simulink model "Clock"  (R2023a)
settings: Solver=VariableStepAuto  StartTime=0.0  StopTime=inf  MaxStep=1  MinStep=1  RelTol=1e-3  EnableMultiTasking=on
libraries: Counters_Lib x14, Nibble_Multiplexers_Lib x9, Bit_Multiplexers_Lib x9, simulink x6, simulink_extras x2, Decoders_Lib x1
settings Model: SimulationMode=accelerator  PauseTimes=0  NumberOfSteps=2  Creator=Jozko Mrkvicka  LastModifiedBy=Jozko Mrkvicka
settings SolverCC: InitialStep=1  AlgebraicLoopSolver=TrustRegion
settings DataIOCC: ReturnWorkspaceOutputs=off
settings OptimizationCC: LifeSpan=inf
settings DebuggingCC: UnconnectedInputMsg=warning  UnconnectedOutputMsg=warning  UnconnectedLineMsg=warning  SFUnexpectedBacktrackingDiag=warning  SFNoUnconditionalDefaultTransitionDiag=warning  ArithmeticOperatorsInVariantConditions=warning
settings ModelReferenceCC: EnableRefExpFcnMdlSchedulingChecks=on
settings SFSimCC: SimUseLocalCustomCode=off  CustomCodeUndefinedFunction=UseInterfaceOnly
settings RTWCC: RTWUseLocalCustomCode=off
settings CodeAppCC: StateflowObjectComments=on
settings GRTTargetCC: TargetLangStandard=C89/C90 (ANSI)
settings ConfigComp: CovMetricSettings=dw  CovSaveCumulativeToWorkspaceVar=on  CovSaveSingleToWorkspaceVar=on  CovExternalEMLEnable=off

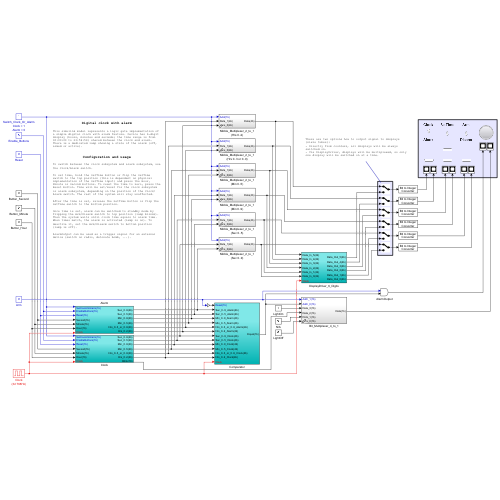
[thumbnail: Simulink's stored preview of the top-level diagram]
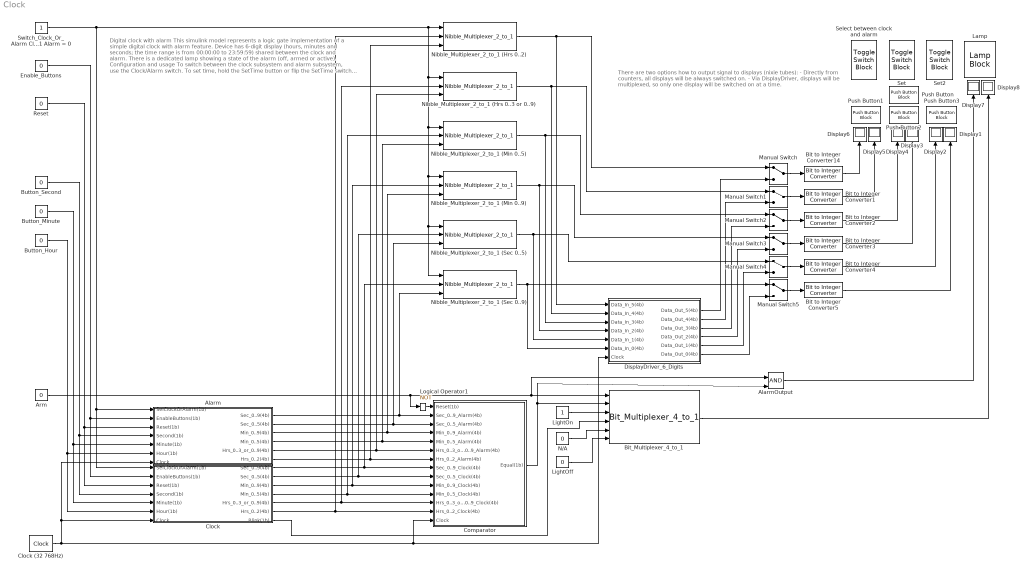
== system Clock ==
  note: There are two options how to output signal to displays (nixie tubes):
      | - Directly from counters, all displays will be always switched on.
      | - Via DisplayDriver, displays will be multiplexed, so only one display will be switched on at a time.
  note: Digital clock with alarm
      |
      | This simulink model represents a logic gate implementation of a simple digital clock with alarm feature. Device has 6-digit display (hours, minutes and seconds; the time range is from 00:00:00 to 23:59:59) shared between the clock and alarm. There is a dedicated lamp showing a state of the alarm (off, armed or active).
      |
      | Configuration and usage
      |
      | To switch between the clock subsystem and alarm subsystem, use the Clock/Alarm switch.
      |
      | To set time, hold the SetTime button or flip the SetTime switch to the top position (this is dependent on physical implementation of the SetTime input) and press the Hour, Minute or Second buttons. To reset the time to zero, press the Reset button. Time will be set/reset for the clock subsystem or alarm subsystem, depending on the position of the Clock/Alarm switch. The rest of the system will stay unaffected.
      |
      | After the time is set, release the SetTime button or flip the SetTime switch to the bottom position.
      |
      | Once time is set, alarm can be switched to standby mode by flipping the Arm/Disarm switch to top position (lamp blinks). Then the system waits until clock time equals to alarm time. When times match, the alarm is activated (lamp is on). To deactive it, set the Arm/Disarm switch to bottom position (lamp is off).
      |
      | AlarmOutput can be used as a trigger signal for an external device (switch on radio, detonate bomb, ...).
  Alarm : Subsystem
  AlarmOutput : Logic  IconShape=distinctive  AllPortsSameDT=off  OutDataTypeStr=boolean
  Arm : Constant  Value=0
  Bit to Integer Converter{1..5,14} (6 alike) : simulink/Logic and Bit Operations/Bit to Integer Converter  nbits=4  bitOrder=MSB first  signedOutputValues=Unsigned  outDtype=uint8  outDtypeSigned=Inherit via internal rule
      settings: LibrarySourceBlock=|
      | commutil2/Bit to Integer
      | Converter
  Bit_Multiplexer_4_to_1 : Bit_Multiplexers_Lib/Bit_Multiplexers_Lib/Bit_Multiplexer_4_to_1  SystemSampleTime=-1  VariantActivationTime=update diagram  Latency=0  AutoFrameSizeCalculation=off
  Button_Hour : Constant  Value=0
  Button_Minute : Constant  Value=0
  Button_Second : Constant  Value=0
  Clock : Subsystem
  Clock (32 768Hz) : simulink_extras/Flip Flops/Clock  period=1
  Comparator : Subsystem
  Display{1..8} (8 alike) : Display
  DisplayDriver_6_Digits : Subsystem
  Enable_Buttons : Constant  Value=0
  Lamp : LampBlock  LabelPosition=Hide
  LightOff : Constant  Value=0
  LightOn : Constant
  Logical Operator1 : Logic  Operator=NOT  Inputs=4  IconShape=distinctive  AllPortsSameDT=off  OutDataTypeStr=boolean
  Manual Switch{,1..5} (6 alike) : ManualSwitch
  N/A : Constant  Value=0
  Nibble_Multiplexer_2_to_1 (Hrs 0..2) : Nibble_Multiplexers_Lib/Nibble_Multiplexers_Lib/Nibble_Multiplexer_2_to_1  SystemSampleTime=-1  VariantActivationTime=update diagram  Latency=0  AutoFrameSizeCalculation=off
  Nibble_Multiplexer_2_to_1 (Hrs 0..3 or 0..9) : Nibble_Multiplexers_Lib/Nibble_Multiplexers_Lib/Nibble_Multiplexer_2_to_1  SystemSampleTime=-1  VariantActivationTime=update diagram  Latency=0  AutoFrameSizeCalculation=off
  Nibble_Multiplexer_2_to_1 (Min 0..5) : Nibble_Multiplexers_Lib/Nibble_Multiplexers_Lib/Nibble_Multiplexer_2_to_1  SystemSampleTime=-1  VariantActivationTime=update diagram  Latency=0  AutoFrameSizeCalculation=off
  Nibble_Multiplexer_2_to_1 (Min 0..9) : Nibble_Multiplexers_Lib/Nibble_Multiplexers_Lib/Nibble_Multiplexer_2_to_1  SystemSampleTime=-1  VariantActivationTime=update diagram  Latency=0  AutoFrameSizeCalculation=off
  Nibble_Multiplexer_2_to_1 (Sec 0..5) : Nibble_Multiplexers_Lib/Nibble_Multiplexers_Lib/Nibble_Multiplexer_2_to_1  SystemSampleTime=-1  VariantActivationTime=update diagram  Latency=0  AutoFrameSizeCalculation=off
  Nibble_Multiplexer_2_to_1 (Sec 0..9) : Nibble_Multiplexers_Lib/Nibble_Multiplexers_Lib/Nibble_Multiplexer_2_to_1  SystemSampleTime=-1  VariantActivationTime=update diagram  Latency=0  AutoFrameSizeCalculation=off
  Push Button : PushButtonBlock  ButtonText=Reset
  Push Button1 : PushButtonBlock  ButtonText=Hour  OffValue=0.000000
  Push Button2 : PushButtonBlock  ButtonText=Minute  OffValue=0.000000
  Push Button3 : PushButtonBlock  ButtonText=Second
  Reset : Constant  Value=0
  Select between clock and alarm : ToggleSwitchBlock  LabelPosition=Hide
      settings: Values={{'Alarm', 'Clock'}, [0 1]}
  Set : ToggleSwitchBlock  LabelPosition=Hide
      settings: Values={{' ', 'SetTime'}, [0 1]}
  Set2 : ToggleSwitchBlock  LabelPosition=Hide
      settings: Values={{'Disarm', 'Arm'}, [0 1]}
  Switch_Clock_Or_Alarm Clock = 1 Alarm = 0 : Constant
  wires:
  Clock (32 768Hz)/1 -> DisplayDriver_6_Digits/7(Clock), Comparator/14(Clock), Clock/7(Clock), Alarm/7(Clock)
  Enable_Buttons/1 -> Clock/2(EnableButtons(1b)), Alarm/2(EnableButtons(1b))
  Reset/1 -> Clock/3(Reset(1b)), Alarm/3(Reset(1b))
  Switch_Clock_Or_Alarm Clock = 1 Alarm = 0/1 -> Nibble_Multiplexer_2_to_1 (Sec 0..9)/1, Nibble_Multiplexer_2_to_1 (Sec 0..5)/1, Nibble_Multiplexer_2_to_1 (Min 0..9)/1, Nibble_Multiplexer_2_to_1 (Min 0..5)/1, Nibble_Multiplexer_2_to_1 (Hrs 0..3 or 0..9)/1, Nibble_Multiplexer_2_to_1 (Hrs 0..2)/1, Clock/1(SelClockOrAlarm(1b)), Alarm/1(SelClockOrAlarm(1b))
  Button_Hour/1 -> Clock/6(Hour(1b)), Alarm/6(Hour(1b))
  Button_Minute/1 -> Clock/5(Minute(1b)), Alarm/5(Minute(1b))
  Button_Second/1 -> Clock/4(Second(1b)), Alarm/4(Second(1b))
  Alarm/6(Hrs_0..2(4b)) -> Nibble_Multiplexer_2_to_1 (Hrs 0..2)/3, Comparator/7(Hrs_0..2_Alarm(4b))
  Alarm/5(Hrs_0..3_or_0..9(4b)) -> Nibble_Multiplexer_2_to_1 (Hrs 0..3 or 0..9)/3, Comparator/6(Hrs_0..3_or_0..9_Alarm(4b))
  Alarm/4(Min_0..5(4b)) -> Nibble_Multiplexer_2_to_1 (Min 0..5)/3, Comparator/5(Min_0..5_Alarm(4b))
  Alarm/3(Min_0..9(4b)) -> Nibble_Multiplexer_2_to_1 (Min 0..9)/3, Comparator/4(Min_0..9_Alarm(4b))
  Alarm/2(Sec_0..5(4b)) -> Nibble_Multiplexer_2_to_1 (Sec 0..5)/3, Comparator/3(Sec_0..5_Alarm(4b))
  Alarm/1(Sec_0..9(4b)) -> Nibble_Multiplexer_2_to_1 (Sec 0..9)/3, Comparator/2(Sec_0..9_Alarm(4b))
  Clock/5(Hrs_0..3_or_0..9(4b)) -> Nibble_Multiplexer_2_to_1 (Hrs 0..3 or 0..9)/2, Comparator/12(Hrs_0..3_or_0..9_Clock(4b))
  Clock/4(Min_0..5(4b)) -> Comparator/11(Min_0..5_Clock(4b)), Nibble_Multiplexer_2_to_1 (Min 0..5)/2
  Clock/3(Min_0..9(4b)) -> Nibble_Multiplexer_2_to_1 (Min 0..9)/2, Comparator/10(Min_0..9_Clock(4b))
  Clock/2(Sec_0..5(4b)) -> Nibble_Multiplexer_2_to_1 (Sec 0..5)/2, Comparator/9(Sec_0..5_Clock(4b))
  Clock/1(Sec_0..9(4b)) -> Nibble_Multiplexer_2_to_1 (Sec 0..9)/2, Comparator/8(Sec_0..9_Clock(4b))
  Clock/6(Hrs_0..2(4b)) -> Nibble_Multiplexer_2_to_1 (Hrs 0..2)/2, Comparator/13(Hrs_0..2_Clock(4b))
  Logical Operator1/1 -> Comparator/1(Reset(1b))
  Arm/1 -> Logical Operator1/1, AlarmOutput/1, Bit_Multiplexer_4_to_1/1
  Comparator/1(Equal(1b)) -> AlarmOutput/2, Bit_Multiplexer_4_to_1/2
  Clock/7(Blink(1b)) -> Bit_Multiplexer_4_to_1/4
  LightOff/1 -> Bit_Multiplexer_4_to_1/6
  LightOn/1 -> Bit_Multiplexer_4_to_1/3
  N/A/1 -> Bit_Multiplexer_4_to_1/5
  Bit_Multiplexer_4_to_1/1 -> Display8/1
  Bit to Integer Converter14/1 -> Display6/1
  Bit to Integer Converter1/1 -> Display5/1
  Bit to Integer Converter2/1 -> Display4/1
  Bit to Integer Converter3/1 -> Display3/1
  Bit to Integer Converter4/1 -> Display2/1
  Bit to Integer Converter5/1 -> Display1/1
  Nibble_Multiplexer_2_to_1 (Hrs 0..2)/1 -> Manual Switch/1, DisplayDriver_6_Digits/1(Data_In_5(4b))
  Nibble_Multiplexer_2_to_1 (Hrs 0..3 or 0..9)/1 -> Manual Switch1/1, DisplayDriver_6_Digits/2(Data_In_4(4b))
  Nibble_Multiplexer_2_to_1 (Min 0..5)/1 -> Manual Switch2/1, DisplayDriver_6_Digits/3(Data_In_3(4b))
  Nibble_Multiplexer_2_to_1 (Min 0..9)/1 -> Manual Switch3/1, DisplayDriver_6_Digits/4(Data_In_2(4b))
  Nibble_Multiplexer_2_to_1 (Sec 0..5)/1 -> Manual Switch4/1, DisplayDriver_6_Digits/5(Data_In_1(4b))
  Nibble_Multiplexer_2_to_1 (Sec 0..9)/1 -> Manual Switch5/1, DisplayDriver_6_Digits/6(Data_In_0(4b))
  DisplayDriver_6_Digits/1(Data_Out_5(4b)) -> Manual Switch/2
  DisplayDriver_6_Digits/2(Data_Out_4(4b)) -> Manual Switch1/2
  DisplayDriver_6_Digits/3(Data_Out_3(4b)) -> Manual Switch2/2
  DisplayDriver_6_Digits/4(Data_Out_2(4b)) -> Manual Switch3/2
  DisplayDriver_6_Digits/5(Data_Out_1(4b)) -> Manual Switch4/2
  DisplayDriver_6_Digits/6(Data_Out_0(4b)) -> Manual Switch5/2
  Manual Switch/1 -> Bit to Integer Converter14/1
  Manual Switch1/1 -> Bit to Integer Converter1/1
  Manual Switch2/1 -> Bit to Integer Converter2/1
  Manual Switch3/1 -> Bit to Integer Converter3/1
  Manual Switch4/1 -> Bit to Integer Converter4/1
  Manual Switch5/1 -> Bit to Integer Converter5/1
  AlarmOutput/1 -> Display7/1

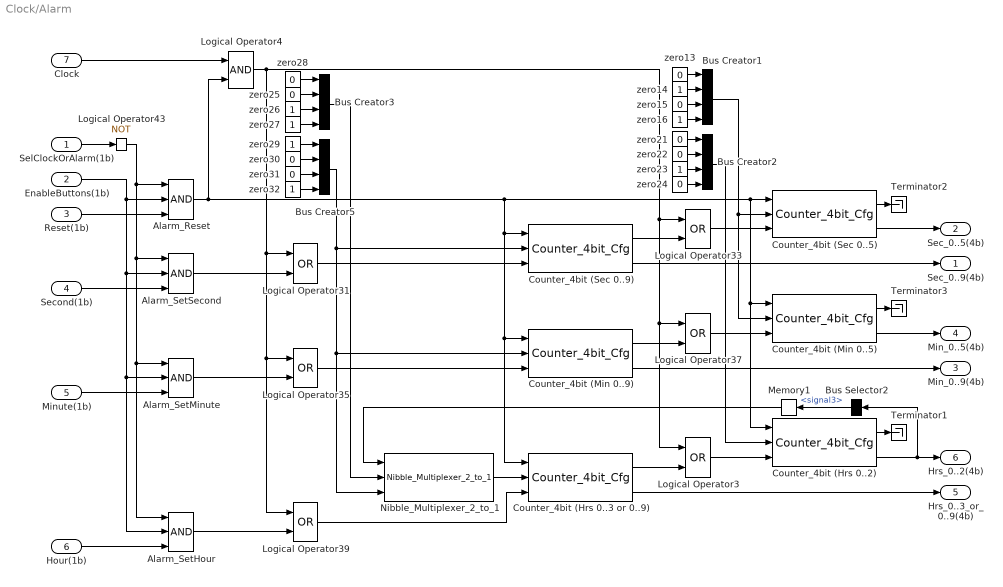
== system Clock/Alarm ==
  SelClockOrAlarm(1b) : Inport
  EnableButtons(1b) : Inport  Port=2
  Reset(1b) : Inport  Port=3
  Second(1b) : Inport  Port=4
  Minute(1b) : Inport  Port=5
  Hour(1b) : Inport  Port=6
  Clock : Inport  Port=7
  Alarm_Reset : Logic  Inputs=3  IconShape=distinctive  AllPortsSameDT=off  OutDataTypeStr=boolean
  Alarm_SetHour : Logic  Inputs=3  IconShape=distinctive  AllPortsSameDT=off  OutDataTypeStr=boolean
  Alarm_SetMinute : Logic  Inputs=3  IconShape=distinctive  AllPortsSameDT=off  OutDataTypeStr=boolean
  Alarm_SetSecond : Logic  Inputs=3  IconShape=distinctive  AllPortsSameDT=off  OutDataTypeStr=boolean
  Bus Creator{1..3,5} (4 alike) : BusCreator  Inputs=4
  Bus Selector2 : BusSelector  OutputSignals=signal3
  Counter_4bit (Hrs 0..3 or 0..9) : Counters_Lib/Counter_4bit_Cfg  SystemSampleTime=-1  VariantActivationTime=update diagram  Latency=0  AutoFrameSizeCalculation=off
  Counter_4bit (Min 0..9) : Counters_Lib/Counter_4bit_Cfg  SystemSampleTime=-1  VariantActivationTime=update diagram  Latency=0  AutoFrameSizeCalculation=off
  Counter_4bit (Sec 0..9) : Counters_Lib/Counter_4bit_Cfg  SystemSampleTime=-1  VariantActivationTime=update diagram  Latency=0  AutoFrameSizeCalculation=off
      settings: LibrarySourceBlock=|
      | Clock_Lib/Counter_4bit
      | (configurable
  Counter_4bit (Hrs 0..2) : Counters_Lib/Counter_4bit_Cfg  SystemSampleTime=-1  VariantActivationTime=update diagram  Latency=0  AutoFrameSizeCalculation=off
  Counter_4bit (Min 0..5) : Counters_Lib/Counter_4bit_Cfg  SystemSampleTime=-1  VariantActivationTime=update diagram  Latency=0  AutoFrameSizeCalculation=off
  Counter_4bit (Sec 0..5) : Counters_Lib/Counter_4bit_Cfg  SystemSampleTime=-1  VariantActivationTime=update diagram  Latency=0  AutoFrameSizeCalculation=off
  Logical Operator{3,31,33,35,37,39} (6 alike) : Logic  Operator=OR  IconShape=distinctive  AllPortsSameDT=off  OutDataTypeStr=boolean
  Logical Operator4 : Logic  IconShape=distinctive  AllPortsSameDT=off  OutDataTypeStr=boolean
  Logical Operator43 : Logic  Operator=NOT  Inputs=4  IconShape=distinctive  AllPortsSameDT=off  OutDataTypeStr=boolean
  Memory1 : Memory
  Nibble_Multiplexer_2_to_1 : Nibble_Multiplexers_Lib/Nibble_Multiplexers_Lib/Nibble_Multiplexer_2_to_1  SystemSampleTime=-1  VariantActivationTime=update diagram  Latency=0  AutoFrameSizeCalculation=off
  Terminator1 : Terminator
  Terminator2 : Terminator
  Terminator3 : Terminator
  zero{13,15,21..22,24..25,28,30..31} (9 alike) : Constant  Value=0
  zero{14,16,23,26..27,29,32} (7 alike) : Constant
  Sec_0..9(4b) : Outport
  Sec_0..5(4b) : Outport  Port=2
  Min_0..9(4b) : Outport  Port=3
  Min_0..5(4b) : Outport  Port=4
  Hrs_0..3_or_0..9(4b) : Outport  Port=5
  Hrs_0..2(4b) : Outport  Port=6
  wires:
  Counter_4bit (Sec 0..9)/1 -> Logical Operator33/2
  Alarm_SetSecond/1 -> Logical Operator31/2
  Alarm_SetMinute/1 -> Logical Operator35/2
  Counter_4bit (Sec 0..9)/2 -> Sec_0..9(4b)/1
  Logical Operator33/1 -> Counter_4bit (Sec 0..5)/3
  Logical Operator31/1 -> Counter_4bit (Sec 0..9)/3
  Alarm_SetHour/1 -> Logical Operator39/2
  Counter_4bit (Min 0..9)/1 -> Logical Operator37/2
  Counter_4bit (Sec 0..5)/2 -> Sec_0..5(4b)/1
  Counter_4bit (Min 0..9)/2 -> Min_0..9(4b)/1
  Logical Operator37/1 -> Counter_4bit (Min 0..5)/3
  Logical Operator43/1 -> Alarm_Reset/1, Alarm_SetSecond/1, Alarm_SetMinute/1, Alarm_SetHour/1
  Logical Operator39/1 -> Counter_4bit (Hrs 0..3 or 0..9)/3
  Logical Operator4/1 -> Logical Operator39/1, Logical Operator35/1, Logical Operator31/1, Logical Operator33/1, Logical Operator37/1, Logical Operator3/1
  Logical Operator35/1 -> Counter_4bit (Min 0..9)/3
  Counter_4bit (Hrs 0..3 or 0..9)/2 -> Hrs_0..3_or_0..9(4b)/1
  Counter_4bit (Hrs 0..2)/2 -> Hrs_0..2(4b)/1, Bus Selector2/1
  Second(1b)/1 -> Alarm_SetSecond/3
  Hour(1b)/1 -> Alarm_SetHour/3
  EnableButtons(1b)/1 -> Alarm_SetHour/2, Alarm_SetMinute/2, Alarm_SetSecond/2, Alarm_Reset/2
  Clock/1 -> Logical Operator4/1
  Reset(1b)/1 -> Alarm_Reset/3
  Minute(1b)/1 -> Alarm_SetMinute/3
  Counter_4bit (Sec 0..5)/1 -> Terminator2/1
  Counter_4bit (Min 0..5)/1 -> Terminator3/1
  Nibble_Multiplexer_2_to_1/1 -> Counter_4bit (Hrs 0..3 or 0..9)/2
  Bus Creator5/1 -> Counter_4bit (Sec 0..9)/2, Counter_4bit (Min 0..9)/2, Nibble_Multiplexer_2_to_1/3
  zero28/1 -> Bus Creator3/1
  zero25/1 -> Bus Creator3/2
  zero26/1 -> Bus Creator3/3
  zero27/1 -> Bus Creator3/4
  Bus Creator3/1 -> Nibble_Multiplexer_2_to_1/2
  zero29/1 -> Bus Creator5/1
  zero30/1 -> Bus Creator5/2
  zero31/1 -> Bus Creator5/3
  zero32/1 -> Bus Creator5/4
  Counter_4bit (Min 0..5)/2 -> Min_0..5(4b)/1
  zero13/1 -> Bus Creator1/1
  zero14/1 -> Bus Creator1/2
  zero15/1 -> Bus Creator1/3
  zero16/1 -> Bus Creator1/4
  Bus Creator1/1 -> Counter_4bit (Min 0..5)/2, Counter_4bit (Sec 0..5)/2
  Memory1/1 -> Nibble_Multiplexer_2_to_1/1
  zero21/1 -> Bus Creator2/1
  zero22/1 -> Bus Creator2/2
  zero23/1 -> Bus Creator2/3
  zero24/1 -> Bus Creator2/4
  Bus Creator2/1 -> Counter_4bit (Hrs 0..2)/2
  Counter_4bit (Hrs 0..2)/1 -> Terminator1/1
  Logical Operator3/1 -> Counter_4bit (Hrs 0..2)/3
  Counter_4bit (Hrs 0..3 or 0..9)/1 -> Logical Operator3/2
  Alarm_Reset/1 -> Logical Operator4/2, Counter_4bit (Sec 0..5)/1, Counter_4bit (Hrs 0..2)/1, Counter_4bit (Min 0..5)/1, Counter_4bit (Sec 0..9)/1, Counter_4bit (Hrs 0..3 or 0..9)/1, Counter_4bit (Min 0..9)/1
  SelClockOrAlarm(1b)/1 -> Logical Operator43/1
  Bus Selector2/1 -> Memory1/1  "<signal3>"

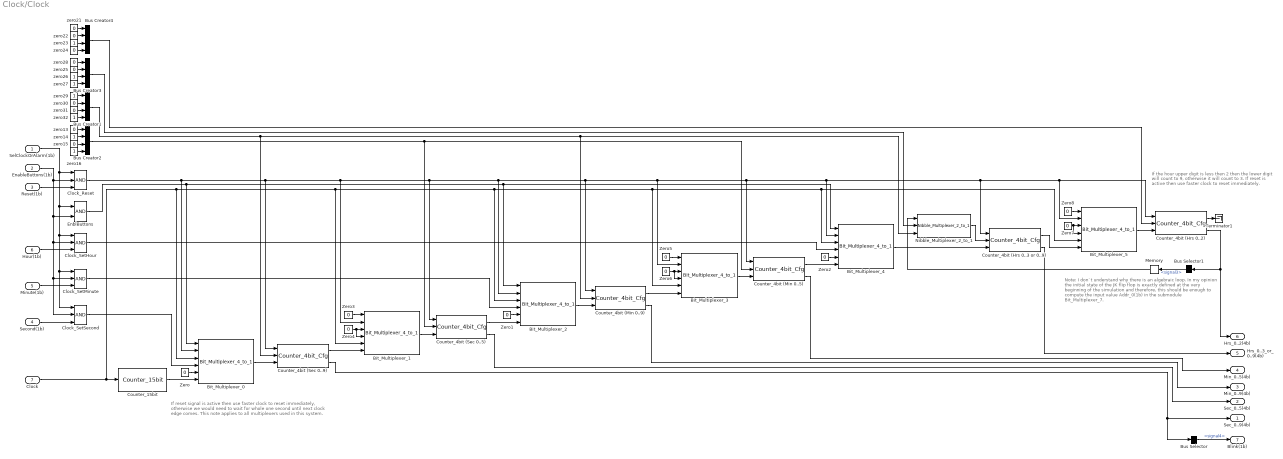
== system Clock/Clock ==
  note: If reset signal is active then use faster clock
      | to reset immediately, otherwise we would need
      | to wait for whole one second until next clock
      | edge comes. This note applies to all multiplexers
      | used in this system.
  note: If the hour upper digit is less then 2
      | then the lower digit will count to 9,
      | otherwise it will count to 3.
      |
      | If reset is active then use faster
      | clock to reset immediately.
  note: Note:
      | I don`t understand why there is an algebraic loop. In my opinion the initial state of the JK flip flop is exactly defined at the very beginning of the simulation and therefore, this should be enough to compute the input value Addr_0(1b) in the submodule Bit_Multiplexer_7.
  SelClockOrAlarm(1b) : Inport
  EnableButtons(1b) : Inport  Port=2
  Reset(1b) : Inport  Port=3
  Second(1b) : Inport  Port=4
  Minute(1b) : Inport  Port=5
  Hour(1b) : Inport  Port=6
  Clock : Inport  Port=7
  Bit_Multiplexer_{0..5} (6 alike) : Bit_Multiplexers_Lib/Bit_Multiplexers_Lib/Bit_Multiplexer_4_to_1  SystemSampleTime=-1  VariantActivationTime=update diagram  Latency=0  AutoFrameSizeCalculation=off
  Bus Creator{1..4} (4 alike) : BusCreator  Inputs=4
  Bus Selector : BusSelector  OutputSignals=signal4
  Bus Selector1 : BusSelector  OutputSignals=signal3
  Clock_Reset : Logic  Inputs=3  IconShape=distinctive  AllPortsSameDT=off  OutDataTypeStr=boolean
  Clock_SetHour : Logic  Inputs=3  IconShape=distinctive  AllPortsSameDT=off  OutDataTypeStr=boolean
  Clock_SetMinute : Logic  Inputs=3  IconShape=distinctive  AllPortsSameDT=off  OutDataTypeStr=boolean
  Clock_SetSecond : Logic  Inputs=3  IconShape=distinctive  AllPortsSameDT=off  OutDataTypeStr=boolean
  Counter_15bit : Counters_Lib/Counter_15bit  SystemSampleTime=-1  VariantActivationTime=update diagram  Latency=0  AutoFrameSizeCalculation=off
  Counter_4bit (Hrs 0..3 or 0..9) : Counters_Lib/Counter_4bit_Cfg  SystemSampleTime=-1  VariantActivationTime=update diagram  Latency=0  AutoFrameSizeCalculation=off
  Counter_4bit (Min 0..9) : Counters_Lib/Counter_4bit_Cfg  SystemSampleTime=-1  VariantActivationTime=update diagram  Latency=0  AutoFrameSizeCalculation=off
  Counter_4bit (Sec 0..9) : Counters_Lib/Counter_4bit_Cfg  SystemSampleTime=-1  VariantActivationTime=update diagram  Latency=0  AutoFrameSizeCalculation=off
  Counter_4bit (Hrs 0..2) : Counters_Lib/Counter_4bit_Cfg  SystemSampleTime=-1  VariantActivationTime=update diagram  Latency=0  AutoFrameSizeCalculation=off
  Counter_4bit (Min 0..5) : Counters_Lib/Counter_4bit_Cfg  SystemSampleTime=-1  VariantActivationTime=update diagram  Latency=0  AutoFrameSizeCalculation=off
  Counter_4bit (Sec 0..5) : Counters_Lib/Counter_4bit_Cfg  SystemSampleTime=-1  VariantActivationTime=update diagram  Latency=0  AutoFrameSizeCalculation=off
  EnblButtons : Logic  IconShape=distinctive  AllPortsSameDT=off  OutDataTypeStr=boolean
  Memory : Memory
  Nibble_Multiplexer_2_to_1 : Nibble_Multiplexers_Lib/Nibble_Multiplexers_Lib/Nibble_Multiplexer_2_to_1  SystemSampleTime=-1  VariantActivationTime=update diagram  Latency=0  AutoFrameSizeCalculation=off
  Terminator1 : Terminator
  Zero{,1..8} (9 alike) : Constant  Value=0
  zero{13,15,21..22,24..25,28,30..31} (9 alike) : Constant  Value=0
  zero{14,16,23,26..27,29,32} (7 alike) : Constant
  Sec_0..9(4b) : Outport
  Sec_0..5(4b) : Outport  Port=2
  Min_0..9(4b) : Outport  Port=3
  Min_0..5(4b) : Outport  Port=4
  Hrs_0..3_or_0..9(4b) : Outport  Port=5
  Hrs_0..2(4b) : Outport  Port=6
  Blink(1b) : Outport  Port=7
  wires:
  Counter_15bit/1 -> Bit_Multiplexer_0/6
  Counter_4bit (Min 0..9)/1 -> Bit_Multiplexer_3/6
  Counter_4bit (Sec 0..9)/1 -> Bit_Multiplexer_1/6
  Bit_Multiplexer_0/1 -> Counter_4bit (Sec 0..9)/3
  Bit_Multiplexer_1/1 -> Counter_4bit (Sec 0..5)/3
  Clock_Reset/1 -> Bit_Multiplexer_0/2, Bit_Multiplexer_1/2, Bit_Multiplexer_2/2, Counter_4bit (Min 0..9)/1, Counter_4bit (Hrs 0..2)/1, Bit_Multiplexer_5/2, Counter_4bit (Hrs 0..3 or 0..9)/1, Bit_Multiplexer_4/2, Counter_4bit (Min 0..5)/1, Bit_Multiplexer_3/2, Counter_4bit (Sec 0..5)/1, Counter_4bit (Sec 0..9)/1
  Counter_4bit (Min 0..5)/1 -> Bit_Multiplexer_4/6
  Clock_SetMinute/1 -> Bit_Multiplexer_2/4
  Clock_SetSecond/1 -> Bit_Multiplexer_0/4
  EnblButtons/1 -> Bit_Multiplexer_0/1, Bit_Multiplexer_2/1, Bit_Multiplexer_4/1
  Clock_SetHour/1 -> Bit_Multiplexer_4/4
  Bit_Multiplexer_2/1 -> Counter_4bit (Min 0..9)/3
  Zero2/1 -> Bit_Multiplexer_4/5
  Zero1/1 -> Bit_Multiplexer_2/5
  Bit_Multiplexer_3/1 -> Counter_4bit (Min 0..5)/3
  Bus Selector1/1 -> Memory/1  "<signal3>"
  Bit_Multiplexer_5/1 -> Counter_4bit (Hrs 0..2)/3
  Bit_Multiplexer_4/1 -> Counter_4bit (Hrs 0..3 or 0..9)/3
  Zero/1 -> Bit_Multiplexer_0/5
  Zero6/1 -> Bit_Multiplexer_3/4, Bit_Multiplexer_3/3
  Zero3/1 -> Bit_Multiplexer_1/1
  Zero4/1 -> Bit_Multiplexer_1/4, Bit_Multiplexer_1/3
  Zero5/1 -> Bit_Multiplexer_3/1
  Counter_4bit (Hrs 0..2)/2 -> Hrs_0..2(4b)/1, Bus Selector1/1
  Hour(1b)/1 -> Clock_SetHour/3
  SelClockOrAlarm(1b)/1 -> Clock_SetSecond/1, Clock_SetMinute/1, Clock_SetHour/1, EnblButtons/1, Clock_Reset/1
  Second(1b)/1 -> Clock_SetSecond/3
  Memory/1 -> Nibble_Multiplexer_2_to_1/1
  Minute(1b)/1 -> Clock_SetMinute/3
  Reset(1b)/1 -> Clock_Reset/3
  Clock/1 -> Counter_15bit/1, Bit_Multiplexer_0/3, Bit_Multiplexer_1/5, Bit_Multiplexer_2/3, Bit_Multiplexer_3/5, Bit_Multiplexer_4/3, Bit_Multiplexer_5/5
  EnableButtons(1b)/1 -> Clock_SetMinute/2, Clock_SetSecond/2, Clock_SetHour/2, EnblButtons/2, Clock_Reset/2
  Counter_4bit (Sec 0..9)/2 -> Bus Selector/1, Sec_0..9(4b)/1
  Bus Selector/1 -> Blink(1b)/1  "<signal4>"
  zero29/1 -> Bus Creator1/1
  zero30/1 -> Bus Creator1/2
  zero31/1 -> Bus Creator1/3
  zero32/1 -> Bus Creator1/4
  Counter_4bit (Min 0..9)/2 -> Min_0..9(4b)/1
  Counter_4bit (Sec 0..5)/1 -> Bit_Multiplexer_2/6
  Counter_4bit (Sec 0..5)/2 -> Sec_0..5(4b)/1
  zero13/1 -> Bus Creator2/1
  zero14/1 -> Bus Creator2/2
  zero15/1 -> Bus Creator2/3
  zero16/1 -> Bus Creator2/4
  Bus Creator2/1 -> Counter_4bit (Sec 0..5)/2, Counter_4bit (Min 0..5)/2
  Counter_4bit (Min 0..5)/2 -> Min_0..5(4b)/1
  Nibble_Multiplexer_2_to_1/1 -> Counter_4bit (Hrs 0..3 or 0..9)/2
  Bus Creator1/1 -> Counter_4bit (Sec 0..9)/2, Counter_4bit (Min 0..9)/2, Nibble_Multiplexer_2_to_1/3
  zero28/1 -> Bus Creator3/1
  zero25/1 -> Bus Creator3/2
  zero26/1 -> Bus Creator3/3
  zero27/1 -> Bus Creator3/4
  Bus Creator3/1 -> Nibble_Multiplexer_2_to_1/2
  Counter_4bit (Hrs 0..3 or 0..9)/1 -> Bit_Multiplexer_5/6
  Counter_4bit (Hrs 0..3 or 0..9)/2 -> Hrs_0..3_or_0..9(4b)/1
  Zero7/1 -> Bit_Multiplexer_5/4, Bit_Multiplexer_5/3
  Zero8/1 -> Bit_Multiplexer_5/1
  Counter_4bit (Hrs 0..2)/1 -> Terminator1/1
  zero21/1 -> Bus Creator4/1
  zero22/1 -> Bus Creator4/2
  zero23/1 -> Bus Creator4/3
  zero24/1 -> Bus Creator4/4
  Bus Creator4/1 -> Counter_4bit (Hrs 0..2)/2

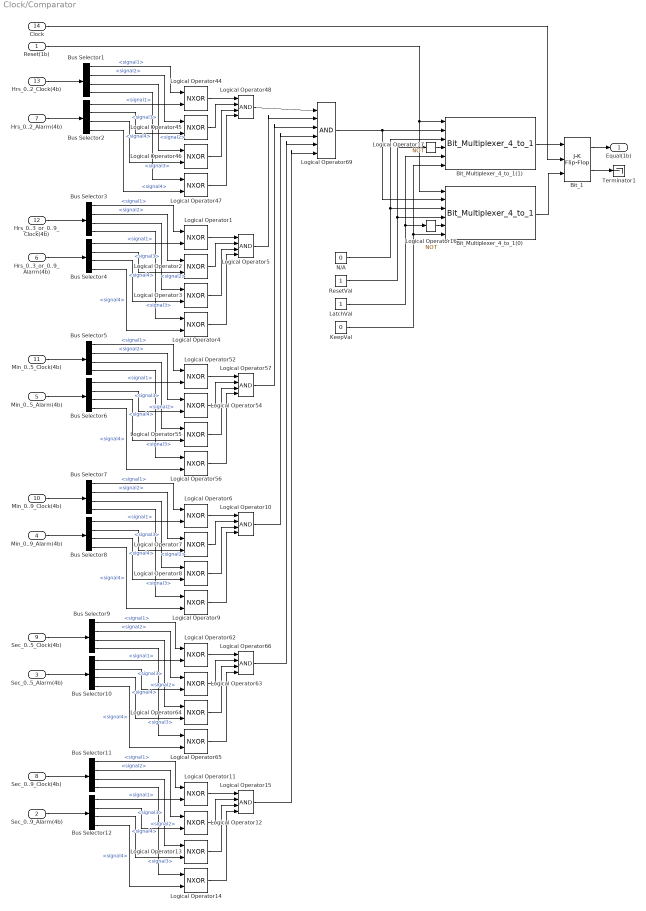
== system Clock/Comparator ==
  Reset(1b) : Inport
  Sec_0..9_Alarm(4b) : Inport  Port=2
  Sec_0..5_Alarm(4b) : Inport  Port=3
  Min_0..9_Alarm(4b) : Inport  Port=4
  Min_0..5_Alarm(4b) : Inport  Port=5
  Hrs_0..3_or_0..9_Alarm(4b) : Inport  Port=6
  Hrs_0..2_Alarm(4b) : Inport  Port=7
  Sec_0..9_Clock(4b) : Inport  Port=8
  Sec_0..5_Clock(4b) : Inport  Port=9
  Min_0..9_Clock(4b) : Inport  Port=10
  Min_0..5_Clock(4b) : Inport  Port=11
  Hrs_0..3_or_0..9_Clock(4b) : Inport  Port=12
  Hrs_0..2_Clock(4b) : Inport  Port=13
  Clock : Inport  Port=14
  Bit_1 : simulink_extras/Flip Flops/J-K Flip-Flop  initial_condition=0
  Bit_Multiplexer_4_to_1(0) : Bit_Multiplexers_Lib/Bit_Multiplexers_Lib/Bit_Multiplexer_4_to_1  SystemSampleTime=-1  VariantActivationTime=update diagram  Latency=0  AutoFrameSizeCalculation=off
  Bit_Multiplexer_4_to_1(1) : Bit_Multiplexers_Lib/Bit_Multiplexers_Lib/Bit_Multiplexer_4_to_1  SystemSampleTime=-1  VariantActivationTime=update diagram  Latency=0  AutoFrameSizeCalculation=off
  Bus Selector{1..12} (12 alike) : BusSelector  OutputSignals=signal1,signal2,signal3,signal4
  KeepVal : Constant  Value=0  OutDataTypeStr=boolean
  LatchVal : Constant  OutDataTypeStr=boolean
  Logical Operator{1..4,6..9,11..14,44..47,52,54..56,62..65} (24 alike) : Logic  Operator=NXOR  IconShape=distinctive  AllPortsSameDT=off  OutDataTypeStr=boolean
  Logical Operator{5,10,15,48,57,66} (6 alike) : Logic  Inputs=4  IconShape=distinctive  AllPortsSameDT=off  OutDataTypeStr=boolean
  Logical Operator16 : Logic  Operator=NOT  Inputs=4  IconShape=distinctive  AllPortsSameDT=off  OutDataTypeStr=boolean
  Logical Operator17 : Logic  Operator=NOT  Inputs=4  IconShape=distinctive  AllPortsSameDT=off  OutDataTypeStr=boolean
  Logical Operator69 : Logic  Inputs=6  IconShape=distinctive  AllPortsSameDT=off  OutDataTypeStr=boolean
  N/A : Constant  Value=0  OutDataTypeStr=boolean
  ResetVal : Constant  OutDataTypeStr=boolean
  Terminator1 : Terminator
  Equal(1b) : Outport
  wires:
  Logical Operator46/1 -> Logical Operator48/3
  Logical Operator15/1 -> Logical Operator69/6
  Logical Operator10/1 -> Logical Operator69/4
  Logical Operator57/1 -> Logical Operator69/3
  Logical Operator44/1 -> Logical Operator48/1
  Logical Operator48/1 -> Logical Operator69/1
  Logical Operator66/1 -> Logical Operator69/5
  Logical Operator55/1 -> Logical Operator57/3
  Logical Operator56/1 -> Logical Operator57/4
  Logical Operator5/1 -> Logical Operator69/2
  Logical Operator69/1 -> Bit_Multiplexer_4_to_1(0)/2, Bit_Multiplexer_4_to_1(1)/2
  Logical Operator47/1 -> Logical Operator48/4
  Logical Operator54/1 -> Logical Operator57/2
  Logical Operator62/1 -> Logical Operator66/1
  Logical Operator63/1 -> Logical Operator66/2
  Logical Operator64/1 -> Logical Operator66/3
  Logical Operator52/1 -> Logical Operator57/1
  Logical Operator45/1 -> Logical Operator48/2
  Logical Operator65/1 -> Logical Operator66/4
  Bus Selector1/1 -> Logical Operator44/1  "<signal1>"
  Bus Selector2/1 -> Logical Operator44/2  "<signal1>"
  Bus Selector1/3 -> Logical Operator46/1  "<signal3>"
  Bus Selector1/4 -> Logical Operator47/1  "<signal4>"
  Bus Selector1/2 -> Logical Operator45/1  "<signal2>"
  Bus Selector2/4 -> Logical Operator47/2  "<signal4>"
  Bus Selector2/2 -> Logical Operator45/2  "<signal2>"
  Logical Operator3/1 -> Logical Operator5/3
  Logical Operator1/1 -> Logical Operator5/1
  Logical Operator4/1 -> Logical Operator5/4
  Logical Operator2/1 -> Logical Operator5/2
  Logical Operator8/1 -> Logical Operator10/3
  Logical Operator6/1 -> Logical Operator10/1
  Logical Operator9/1 -> Logical Operator10/4
  Logical Operator7/1 -> Logical Operator10/2
  Logical Operator13/1 -> Logical Operator15/3
  Logical Operator11/1 -> Logical Operator15/1
  Logical Operator14/1 -> Logical Operator15/4
  Logical Operator12/1 -> Logical Operator15/2
  Bus Selector2/3 -> Logical Operator46/2  "<signal3>"
  Bus Selector3/1 -> Logical Operator1/1  "<signal1>"
  Bus Selector4/1 -> Logical Operator1/2  "<signal1>"
  Bus Selector3/3 -> Logical Operator3/1  "<signal3>"
  Bus Selector3/4 -> Logical Operator4/1  "<signal4>"
  Bus Selector3/2 -> Logical Operator2/1  "<signal2>"
  Bus Selector4/4 -> Logical Operator4/2  "<signal4>"
  Bus Selector4/2 -> Logical Operator2/2  "<signal2>"
  Bus Selector4/3 -> Logical Operator3/2  "<signal3>"
  Bus Selector5/1 -> Logical Operator52/1  "<signal1>"
  Bus Selector6/1 -> Logical Operator52/2  "<signal1>"
  Bus Selector5/3 -> Logical Operator55/1  "<signal3>"
  Bus Selector5/4 -> Logical Operator56/1  "<signal4>"
  Bus Selector5/2 -> Logical Operator54/1  "<signal2>"
  Bus Selector6/4 -> Logical Operator56/2  "<signal4>"
  Bus Selector6/2 -> Logical Operator54/2  "<signal2>"
  Bus Selector6/3 -> Logical Operator55/2  "<signal3>"
  Bus Selector7/1 -> Logical Operator6/1  "<signal1>"
  Bus Selector8/1 -> Logical Operator6/2  "<signal1>"
  Bus Selector7/3 -> Logical Operator8/1  "<signal3>"
  Bus Selector7/4 -> Logical Operator9/1  "<signal4>"
  Bus Selector7/2 -> Logical Operator7/1  "<signal2>"
  Bus Selector8/4 -> Logical Operator9/2  "<signal4>"
  Bus Selector8/2 -> Logical Operator7/2  "<signal2>"
  Bus Selector8/3 -> Logical Operator8/2  "<signal3>"
  Bus Selector9/1 -> Logical Operator62/1  "<signal1>"
  Bus Selector10/1 -> Logical Operator62/2  "<signal1>"
  Bus Selector9/3 -> Logical Operator64/1  "<signal3>"
  Bus Selector9/4 -> Logical Operator65/1  "<signal4>"
  Bus Selector9/2 -> Logical Operator63/1  "<signal2>"
  Bus Selector10/4 -> Logical Operator65/2  "<signal4>"
  Bus Selector10/2 -> Logical Operator63/2  "<signal2>"
  Bus Selector10/3 -> Logical Operator64/2  "<signal3>"
  Bus Selector11/1 -> Logical Operator11/1  "<signal1>"
  Bus Selector12/1 -> Logical Operator11/2  "<signal1>"
  Bus Selector11/3 -> Logical Operator13/1  "<signal3>"
  Bus Selector11/4 -> Logical Operator14/1  "<signal4>"
  Bus Selector11/2 -> Logical Operator12/1  "<signal2>"
  Bus Selector12/4 -> Logical Operator14/2  "<signal4>"
  Bus Selector12/2 -> Logical Operator12/2  "<signal2>"
  Bus Selector12/3 -> Logical Operator13/2  "<signal3>"
  Hrs_0..2_Clock(4b)/1 -> Bus Selector1/1
  Hrs_0..2_Alarm(4b)/1 -> Bus Selector2/1
  Hrs_0..3_or_0..9_Clock(4b)/1 -> Bus Selector3/1
  Hrs_0..3_or_0..9_Alarm(4b)/1 -> Bus Selector4/1
  Min_0..5_Clock(4b)/1 -> Bus Selector5/1
  Min_0..5_Alarm(4b)/1 -> Bus Selector6/1
  Min_0..9_Clock(4b)/1 -> Bus Selector7/1
  Min_0..9_Alarm(4b)/1 -> Bus Selector8/1
  Sec_0..5_Clock(4b)/1 -> Bus Selector9/1
  Sec_0..5_Alarm(4b)/1 -> Bus Selector10/1
  Sec_0..9_Clock(4b)/1 -> Bus Selector11/1
  Sec_0..9_Alarm(4b)/1 -> Bus Selector12/1
  Reset(1b)/1 -> Bit_Multiplexer_4_to_1(0)/1, Bit_Multiplexer_4_to_1(1)/1
  Bit_1/1 -> Equal(1b)/1
  Bit_1/2 -> Terminator1/1
  Bit_Multiplexer_4_to_1(0)/1 -> Bit_1/3
  Bit_Multiplexer_4_to_1(1)/1 -> Bit_1/1
  KeepVal/1 -> Bit_Multiplexer_4_to_1(1)/6, Bit_Multiplexer_4_to_1(0)/6
  LatchVal/1 -> Bit_Multiplexer_4_to_1(1)/5, Logical Operator16/1
  Logical Operator16/1 -> Bit_Multiplexer_4_to_1(0)/5
  ResetVal/1 -> Logical Operator17/1, Bit_Multiplexer_4_to_1(0)/4
  N/A/1 -> Bit_Multiplexer_4_to_1(1)/3, Bit_Multiplexer_4_to_1(0)/3
  Clock/1 -> Bit_1/2
  Logical Operator17/1 -> Bit_Multiplexer_4_to_1(1)/4

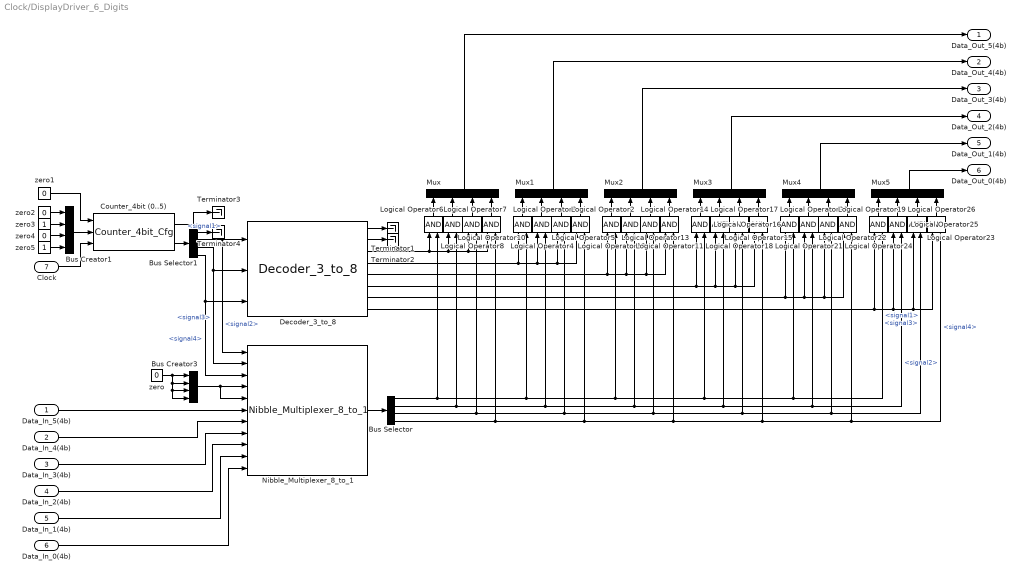
== system Clock/DisplayDriver_6_Digits ==
  Data_In_5(4b) : Inport
  Data_In_4(4b) : Inport  Port=2
  Data_In_3(4b) : Inport  Port=3
  Data_In_2(4b) : Inport  Port=4
  Data_In_1(4b) : Inport  Port=5
  Data_In_0(4b) : Inport  Port=6
  Clock : Inport  Port=7
  Bus Creator1 : BusCreator  Inputs=4
  Bus Creator3 : BusCreator  Inputs=4
  Bus Selector : BusSelector  OutputSignals=signal1,signal2,signal3,signal4
  Bus Selector1 : BusSelector  OutputSignals=signal1,signal2,signal3,signal4
  Counter_4bit (0..5) : Counters_Lib/Counter_4bit_Cfg  SystemSampleTime=-1  VariantActivationTime=update diagram  Latency=0  AutoFrameSizeCalculation=off
  Decoder_3_to_8 : Decoders_Lib/Decoders_Lib/Decoder_3_to_8  SystemSampleTime=-1  VariantActivationTime=update diagram  Latency=0  AutoFrameSizeCalculation=off
  Logical Operator{2..8,10..26} (24 alike) : Logic  IconShape=distinctive  AllPortsSameDT=off  OutDataTypeStr=boolean
  Mux{,1..5} (6 alike) : Mux
  Nibble_Multiplexer_8_to_1 : Nibble_Multiplexers_Lib/Nibble_Multiplexers_Lib/Nibble_Multiplexer_8_to_1  SystemSampleTime=-1  VariantActivationTime=update diagram  Latency=0  AutoFrameSizeCalculation=off
  Terminator{1..4} (4 alike) : Terminator
  zero{,1..2,4} (4 alike) : Constant  Value=0
  zero3 : Constant
  zero5 : Constant
  Data_Out_5(4b) : Outport
  Data_Out_4(4b) : Outport  Port=2
  Data_Out_3(4b) : Outport  Port=3
  Data_Out_2(4b) : Outport  Port=4
  Data_Out_1(4b) : Outport  Port=5
  Data_Out_0(4b) : Outport  Port=6
  wires:
  Data_In_4(4b)/1 -> Nibble_Multiplexer_8_to_1/7
  Data_In_3(4b)/1 -> Nibble_Multiplexer_8_to_1/8
  Data_In_2(4b)/1 -> Nibble_Multiplexer_8_to_1/9
  Data_In_1(4b)/1 -> Nibble_Multiplexer_8_to_1/10
  zero/1 -> Bus Creator3/4, Bus Creator3/3, Bus Creator3/2, Bus Creator3/1
  Bus Creator3/1 -> Nibble_Multiplexer_8_to_1/5, Nibble_Multiplexer_8_to_1/4
  Bus Selector1/4 -> Nibble_Multiplexer_8_to_1/3, Decoder_3_to_8/3  "<signal4>"
  Data_In_0(4b)/1 -> Nibble_Multiplexer_8_to_1/11
  Nibble_Multiplexer_8_to_1/1 -> Bus Selector/1
  Bus Selector1/3 -> Decoder_3_to_8/2, Nibble_Multiplexer_8_to_1/2  "<signal3>"
  Decoder_3_to_8/3 -> Logical Operator6/1, Logical Operator7/1, Logical Operator8/1, Logical Operator10/1
  Decoder_3_to_8/1 -> Terminator1/1
  Decoder_3_to_8/2 -> Terminator2/1
  Data_In_5(4b)/1 -> Nibble_Multiplexer_8_to_1/6
  Mux3/1 -> Data_Out_2(4b)/1
  Logical Operator5/1 -> Mux1/3
  Logical Operator2/1 -> Mux1/4
  Logical Operator3/1 -> Mux1/1
  Logical Operator4/1 -> Mux1/2
  Bus Selector1/2 -> Decoder_3_to_8/1, Nibble_Multiplexer_8_to_1/1  "<signal2>"
  Mux/1 -> Data_Out_5(4b)/1
  Decoder_3_to_8/6 -> Logical Operator16/1, Logical Operator17/1, Logical Operator18/1, Logical Operator15/1
  Decoder_3_to_8/8 -> Logical Operator24/1, Logical Operator25/1, Logical Operator26/1, Logical Operator23/1
  Logical Operator19/1 -> Mux4/4
  Logical Operator22/1 -> Mux4/3
  Logical Operator20/1 -> Mux4/1
  Logical Operator21/1 -> Mux4/2
  Bus Selector/1 -> Logical Operator6/2, Logical Operator24/2, Logical Operator20/2, Logical Operator16/2, Logical Operator12/2, Logical Operator3/2  "<signal1>"
  Decoder_3_to_8/4 -> Logical Operator3/1, Logical Operator4/1, Logical Operator5/1, Logical Operator2/1
  Mux4/1 -> Data_Out_1(4b)/1
  Mux5/1 -> Data_Out_0(4b)/1
  Decoder_3_to_8/7 -> Logical Operator20/1, Logical Operator21/1, Logical Operator22/1, Logical Operator19/1
  Decoder_3_to_8/5 -> Logical Operator12/1, Logical Operator13/1, Logical Operator14/1, Logical Operator11/1
  Mux1/1 -> Data_Out_4(4b)/1
  Mux2/1 -> Data_Out_3(4b)/1
  Logical Operator17/1 -> Mux3/2
  Logical Operator18/1 -> Mux3/3
  Logical Operator16/1 -> Mux3/1
  Logical Operator15/1 -> Mux3/4
  Bus Selector/2 -> Logical Operator7/2, Logical Operator25/2, Logical Operator21/2, Logical Operator17/2, Logical Operator13/2, Logical Operator4/2  "<signal2>"
  Bus Selector/4 -> Logical Operator10/2, Logical Operator23/2, Logical Operator19/2, Logical Operator15/2, Logical Operator11/2, Logical Operator2/2  "<signal4>"
  Logical Operator14/1 -> Mux2/3
  Logical Operator11/1 -> Mux2/4
  Logical Operator25/1 -> Mux5/2
  Logical Operator23/1 -> Mux5/4
  Logical Operator12/1 -> Mux2/1
  Logical Operator7/1 -> Mux/2
  Logical Operator6/1 -> Mux/1
  Logical Operator26/1 -> Mux5/3
  Logical Operator13/1 -> Mux2/2
  Logical Operator24/1 -> Mux5/1
  Bus Selector/3 -> Logical Operator8/2, Logical Operator22/2, Logical Operator26/2, Logical Operator18/2, Logical Operator14/2, Logical Operator5/2  "<signal3>"
  Logical Operator8/1 -> Mux/3
  Logical Operator10/1 -> Mux/4
  Counter_4bit (0..5)/1 -> Terminator3/1
  zero1/1 -> Counter_4bit (0..5)/1
  zero2/1 -> Bus Creator1/1
  zero3/1 -> Bus Creator1/2
  zero4/1 -> Bus Creator1/3
  zero5/1 -> Bus Creator1/4
  Bus Creator1/1 -> Counter_4bit (0..5)/2
  Clock/1 -> Counter_4bit (0..5)/3
  Counter_4bit (0..5)/2 -> Bus Selector1/1
  Bus Selector1/1 -> Terminator4/1  "<signal1>"
